simulink model "BD_DynamicCompareSims2"  (Simulink 4.1.1)
settings: Solver=VariableStepDiscrete  StartTime=0.0  StopTime=inf  FixedStep=1  RelTol=1e-3
undefined symbols (not defined in the file or in its folder): ALTIAHOME, cyc_mph_r1, ess_pwr_out_a1, ess_pwr_out_a2, ess_soc_hist1, ess_soc_hist2, fc_brake_trq1, fc_brake_trq2, fc_eff_out_a1, fc_eff_out_a2, fc_fuel_rate1, fc_fuel_rate2, fc_pwr_out_a1, fc_pwr_out_a2, fc_spd_est1, fc_spd_est2, gal1, gal2, gc_pwr_out_a1, gc_pwr_out_a2, gear_number1, gear_number2, grade1, grade2, mc_spd_out_a1, mc_spd_out_a2, mc_trq_out_a1, mc_trq_out_a2, mpha1, mpha2, time1, time2, trace_miss1, trace_miss2, veh_pwr_accel_a1, veh_pwr_accel_a2, veh_pwr_ascent_a1, veh_pwr_ascent_a2, veh_pwr_drag_a1, veh_pwr_drag_a2, veh_pwr_rr_a1, veh_pwr_rr_a2
libraries: simulink3 x4
settings Model: LastModifiedBy=abrooker

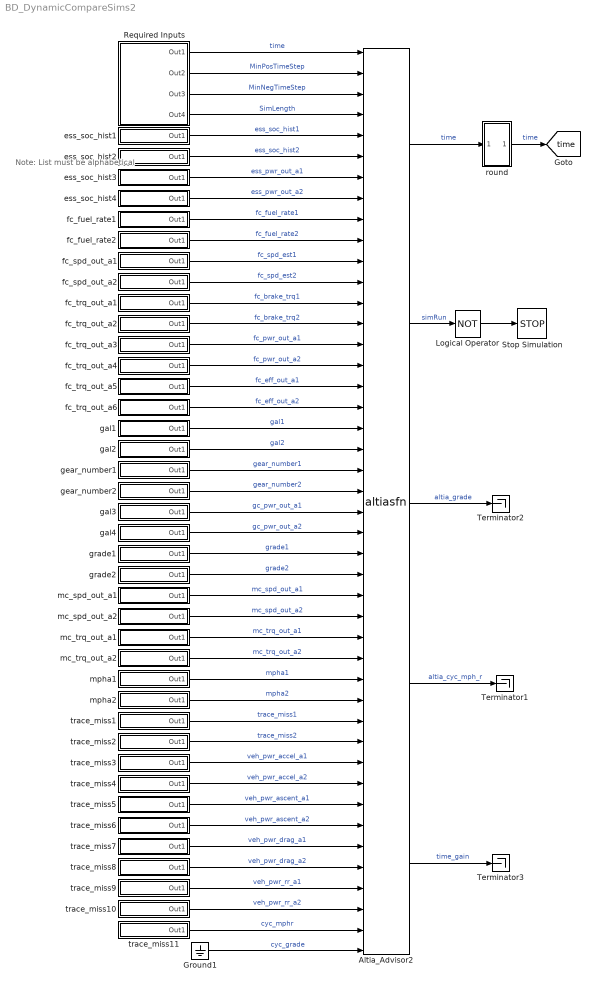
== system BD_DynamicCompareSims2 ==
  note: Note:  List must
      | be alphabetical
  Altia_Advisor2 : S-Function  FunctionName=altiasfn  Parameters=NumAltiaSfnInputs,NumAltiaSfnOutputs,ALTIAHOME  PortCounts=[]  SFunctionModules=libsdde.lib user32.lib  mask{NumAltiaSfnInputs=44, NumAltiaSfnOutputs=5}
      mask prompts: NumAltiaSfnInputs "Inputs to Altia S-Function:"; NumAltiaSfnOutputs "Outputs to Altia S-Function:"
      mask help: This block allows you to connect your signals to an Altia Design file. Specify the number of Inputs and Outputs you would like the Altia block to have (each line connected to the block can only be ONE signal wide ... no muxing into the Altia block).
      mask init:
      | altiahome
      settings: OpenFcn=AltiaClk
      mask Help: The first box is the number of inputs to the Altia S-Function.  The second box is the number of ouputs for the Altia S-Function.
      mask Display: disp('A L T I A')
  Ground1 : Ground
  Logical Operator : Logic  Operator=NOT  Inputs=2
  Required Inputs : Subsystem
      settings: RTWFcnNameOpts=Auto  RTWFileNameOpts=Auto
      mask Display: disp('Required Inputs');
  Stop Simulation : Stop
  Terminator1 : Terminator
  Terminator2 : Terminator
  Terminator3 : Terminator
  ess_soc_hist1 : Subsystem  mask{outputVector=ess_soc_hist1, timeVector=time1}
      mask prompts: outputVector "Output"; timeVector "Time Vector"
      settings: RTWFcnNameOpts=Auto  RTWFileNameOpts=Auto
      mask Display: disp('');
  ess_soc_hist2 : Subsystem  mask{outputVector=ess_soc_hist2, timeVector=time2}
      mask prompts: outputVector "Output"; timeVector "Time Vector"
      settings: RTWFcnNameOpts=Auto  RTWFileNameOpts=Auto
      mask Display: disp('');
  ess_soc_hist3 : Subsystem  mask{outputVector=ess_pwr_out_a1, timeVector=time1}
      mask prompts: outputVector "Output"; timeVector "Time Vector"
      settings: RTWFcnNameOpts=Auto  RTWFileNameOpts=Auto
      mask Display: disp('');
  ess_soc_hist4 : Subsystem  mask{outputVector=ess_pwr_out_a2, timeVector=time2}
      mask prompts: outputVector "Output"; timeVector "Time Vector"
      settings: RTWFcnNameOpts=Auto  RTWFileNameOpts=Auto
      mask Display: disp('');
  fc_fuel_rate1 : Subsystem  mask{outputVector=fc_fuel_rate1, timeVector=time1}
      mask prompts: outputVector "Output"; timeVector "Time Vector"
      settings: RTWFcnNameOpts=Auto  RTWFileNameOpts=Auto
      mask Display: disp('');
  fc_fuel_rate2 : Subsystem  mask{outputVector=fc_fuel_rate2, timeVector=time2}
      mask prompts: outputVector "Output"; timeVector "Time Vector"
      settings: RTWFcnNameOpts=Auto  RTWFileNameOpts=Auto
      mask Display: disp('');
  fc_spd_out_a1 : Subsystem  mask{outputVector=fc_spd_est1, timeVector=time1}
      mask prompts: outputVector "Output"; timeVector "Time Vector"
      settings: RTWFcnNameOpts=Auto  RTWFileNameOpts=Auto
      mask Display: disp('');
  fc_spd_out_a2 : Subsystem  mask{outputVector=fc_spd_est2, timeVector=time2}
      mask prompts: outputVector "Output"; timeVector "Time Vector"
      settings: RTWFcnNameOpts=Auto  RTWFileNameOpts=Auto
      mask Display: disp('');
  fc_trq_out_a1 : Subsystem  mask{outputVector=fc_brake_trq1, timeVector=time1}
      mask prompts: outputVector "Output"; timeVector "Time Vector"
      settings: RTWFcnNameOpts=Auto  RTWFileNameOpts=Auto
      mask Display: disp('');
  fc_trq_out_a2 : Subsystem  mask{outputVector=fc_brake_trq2, timeVector=time2}
      mask prompts: outputVector "Output"; timeVector "Time Vector"
      settings: RTWFcnNameOpts=Auto  RTWFileNameOpts=Auto
      mask Display: disp('');
  fc_trq_out_a3 : Subsystem  mask{outputVector=fc_pwr_out_a1, timeVector=time1}
      mask prompts: outputVector "Output"; timeVector "Time Vector"
      settings: RTWFcnNameOpts=Auto  RTWFileNameOpts=Auto
      mask Display: disp('');
  fc_trq_out_a4 : Subsystem  mask{outputVector=fc_pwr_out_a2, timeVector=time2}
      mask prompts: outputVector "Output"; timeVector "Time Vector"
      settings: RTWFcnNameOpts=Auto  RTWFileNameOpts=Auto
      mask Display: disp('');
  fc_trq_out_a5 : Subsystem  mask{outputVector=fc_eff_out_a1, timeVector=time1}
      mask prompts: outputVector "Output"; timeVector "Time Vector"
      settings: RTWFcnNameOpts=Auto  RTWFileNameOpts=Auto
      mask Display: disp('');
  fc_trq_out_a6 : Subsystem  mask{outputVector=fc_eff_out_a2, timeVector=time2}
      mask prompts: outputVector "Output"; timeVector "Time Vector"
      settings: RTWFcnNameOpts=Auto  RTWFileNameOpts=Auto
      mask Display: disp('');
  gal1 : Subsystem  mask{outputVector=gal1, timeVector=time1}
      mask prompts: outputVector "Output"; timeVector "Time Vector"
      settings: RTWFcnNameOpts=Auto  RTWFileNameOpts=Auto
      mask Display: disp('');
  gal2 : Subsystem  mask{outputVector=gal2, timeVector=time2}
      mask prompts: outputVector "Output"; timeVector "Time Vector"
      settings: RTWFcnNameOpts=Auto  RTWFileNameOpts=Auto
      mask Display: disp('');
  gal3 : Subsystem  mask{outputVector=gc_pwr_out_a1, timeVector=time1}
      mask prompts: outputVector "Output"; timeVector "Time Vector"
      settings: RTWFcnNameOpts=Auto  RTWFileNameOpts=Auto
      mask Display: disp('');
  gal4 : Subsystem  mask{outputVector=gc_pwr_out_a2, timeVector=time2}
      mask prompts: outputVector "Output"; timeVector "Time Vector"
      settings: RTWFcnNameOpts=Auto  RTWFileNameOpts=Auto
      mask Display: disp('');
  gear_number1 : Subsystem  mask{outputVector=gear_number1, timeVector=time1}
      mask prompts: outputVector "Output"; timeVector "Time Vector"
      settings: RTWFcnNameOpts=Auto  RTWFileNameOpts=Auto
      mask Display: disp('');
  gear_number2 : Subsystem  mask{outputVector=gear_number2, timeVector=time2}
      mask prompts: outputVector "Output"; timeVector "Time Vector"
      settings: RTWFcnNameOpts=Auto  RTWFileNameOpts=Auto
      mask Display: disp('');
  grade1 : Subsystem  mask{outputVector=grade1, timeVector=time1}
      mask prompts: outputVector "Output"; timeVector "Time Vector"
      settings: RTWFcnNameOpts=Auto  RTWFileNameOpts=Auto
      mask Display: disp('');
  grade2 : Subsystem  mask{outputVector=grade2, timeVector=time2}
      mask prompts: outputVector "Output"; timeVector "Time Vector"
      settings: RTWFcnNameOpts=Auto  RTWFileNameOpts=Auto
      mask Display: disp('');
  mc_spd_out_a1 : Subsystem  mask{outputVector=mc_spd_out_a1, timeVector=time1}
      mask prompts: outputVector "Output"; timeVector "Time Vector"
      settings: RTWFcnNameOpts=Auto  RTWFileNameOpts=Auto
      mask Display: disp('');
  mc_spd_out_a2 : Subsystem  mask{outputVector=mc_spd_out_a2, timeVector=time2}
      mask prompts: outputVector "Output"; timeVector "Time Vector"
      settings: RTWFcnNameOpts=Auto  RTWFileNameOpts=Auto
      mask Display: disp('');
  mc_trq_out_a1 : Subsystem  mask{outputVector=mc_trq_out_a1, timeVector=time1}
      mask prompts: outputVector "Output"; timeVector "Time Vector"
      settings: RTWFcnNameOpts=Auto  RTWFileNameOpts=Auto
      mask Display: disp('');
  mc_trq_out_a2 : Subsystem  mask{outputVector=mc_trq_out_a2, timeVector=time2}
      mask prompts: outputVector "Output"; timeVector "Time Vector"
      settings: RTWFcnNameOpts=Auto  RTWFileNameOpts=Auto
      mask Display: disp('');
  mpha1 : Subsystem  mask{outputVector=mpha1, timeVector=time1}
      mask prompts: outputVector "Output"; timeVector "Time Vector"
      settings: RTWFcnNameOpts=Auto  RTWFileNameOpts=Auto
      mask Display: disp('');
  mpha2 : Subsystem  mask{outputVector=mpha2, timeVector=time2}
      mask prompts: outputVector "Output"; timeVector "Time Vector"
      settings: RTWFcnNameOpts=Auto  RTWFileNameOpts=Auto
      mask Display: disp('');
  round : Subsystem  mask{DecPlace=.001}
      mask prompts: DecPlace "Decimal Place (Example:  .001 rounds 1.2222 to 1.2200)"
      settings: RTWFcnNameOpts=Auto  RTWFileNameOpts=Auto
  trace_miss1 : Subsystem  mask{outputVector=trace_miss1, timeVector=time1}
      mask prompts: outputVector "Output"; timeVector "Time Vector"
      settings: RTWFcnNameOpts=Auto  RTWFileNameOpts=Auto
      mask Display: disp('');
  trace_miss10 : Subsystem  mask{outputVector=veh_pwr_rr_a2, timeVector=time2}
      mask prompts: outputVector "Output"; timeVector "Time Vector"
      settings: RTWFcnNameOpts=Auto  RTWFileNameOpts=Auto
      mask Display: disp('');
  trace_miss11 : Subsystem  mask{outputVector=cyc_mph_r1, timeVector=time1}
      mask prompts: outputVector "Output"; timeVector "Time Vector"
      settings: RTWFcnNameOpts=Auto  RTWFileNameOpts=Auto
      mask Display: disp('');
  trace_miss2 : Subsystem  mask{outputVector=trace_miss2, timeVector=time2}
      mask prompts: outputVector "Output"; timeVector "Time Vector"
      settings: RTWFcnNameOpts=Auto  RTWFileNameOpts=Auto
      mask Display: disp('');
  trace_miss3 : Subsystem  mask{outputVector=veh_pwr_accel_a1, timeVector=time1}
      mask prompts: outputVector "Output"; timeVector "Time Vector"
      settings: RTWFcnNameOpts=Auto  RTWFileNameOpts=Auto
      mask Display: disp('');
  trace_miss4 : Subsystem  mask{outputVector=veh_pwr_accel_a2, timeVector=time2}
      mask prompts: outputVector "Output"; timeVector "Time Vector"
      settings: RTWFcnNameOpts=Auto  RTWFileNameOpts=Auto
      mask Display: disp('');
  trace_miss5 : Subsystem  mask{outputVector=veh_pwr_ascent_a1, timeVector=time1}
      mask prompts: outputVector "Output"; timeVector "Time Vector"
      settings: RTWFcnNameOpts=Auto  RTWFileNameOpts=Auto
      mask Display: disp('');
  trace_miss6 : Subsystem  mask{outputVector=veh_pwr_ascent_a2, timeVector=time2}
      mask prompts: outputVector "Output"; timeVector "Time Vector"
      settings: RTWFcnNameOpts=Auto  RTWFileNameOpts=Auto
      mask Display: disp('');
  trace_miss7 : Subsystem  mask{outputVector=veh_pwr_drag_a1, timeVector=time1}
      mask prompts: outputVector "Output"; timeVector "Time Vector"
      settings: RTWFcnNameOpts=Auto  RTWFileNameOpts=Auto
      mask Display: disp('');
  trace_miss8 : Subsystem  mask{outputVector=veh_pwr_drag_a2, timeVector=time2}
      mask prompts: outputVector "Output"; timeVector "Time Vector"
      settings: RTWFcnNameOpts=Auto  RTWFileNameOpts=Auto
      mask Display: disp('');
  trace_miss9 : Subsystem  mask{outputVector=veh_pwr_rr_a1, timeVector=time1}
      mask prompts: outputVector "Output"; timeVector "Time Vector"
      settings: RTWFcnNameOpts=Auto  RTWFileNameOpts=Auto
      mask Display: disp('');
  tag scope: time=global
  wires:
  Altia_Advisor2/1 -> round/1(In1)  "time"
  Required Inputs/2(Out2) -> Altia_Advisor2/2  "MinPosTimeStep"
  Required Inputs/3(Out3) -> Altia_Advisor2/3  "MinNegTimeStep"
  Required Inputs/4(Out4) -> Altia_Advisor2/4  "SimLength"
  Required Inputs/1(Out1) -> Altia_Advisor2/1  "time"
  round/1(Out1) -> [time]  "time"
  Altia_Advisor2/2 -> Logical Operator/1  "simRun"
  ess_soc_hist1/1(Out1) -> Altia_Advisor2/5  "ess_soc_hist1"
  ess_soc_hist2/1(Out1) -> Altia_Advisor2/6  "ess_soc_hist2"
  fc_fuel_rate2/1(Out1) -> Altia_Advisor2/10  "fc_fuel_rate2"
  fc_spd_out_a1/1(Out1) -> Altia_Advisor2/11  "fc_spd_est1"
  fc_spd_out_a2/1(Out1) -> Altia_Advisor2/12  "fc_spd_est2"
  fc_trq_out_a1/1(Out1) -> Altia_Advisor2/13  "fc_brake_trq1"
  fc_trq_out_a2/1(Out1) -> Altia_Advisor2/14  "fc_brake_trq2"
  Altia_Advisor2/3 -> Terminator2/1  "altia_grade"
  Altia_Advisor2/4 -> Terminator1/1  "altia_cyc_mph_r"
  Altia_Advisor2/5 -> Terminator3/1  "time_gain"
  fc_trq_out_a3/1(Out1) -> Altia_Advisor2/15  "fc_pwr_out_a1"
  gal1/1(Out1) -> Altia_Advisor2/19  "gal1"
  gal2/1(Out1) -> Altia_Advisor2/20  "gal2"
  gear_number1/1(Out1) -> Altia_Advisor2/21  "gear_number1"
  gear_number2/1(Out1) -> Altia_Advisor2/22  "gear_number2"
  grade1/1(Out1) -> Altia_Advisor2/25  "grade1"
  grade2/1(Out1) -> Altia_Advisor2/26  "grade2"
  mc_spd_out_a1/1(Out1) -> Altia_Advisor2/27  "mc_spd_out_a1"
  mc_spd_out_a2/1(Out1) -> Altia_Advisor2/28  "mc_spd_out_a2"
  mc_trq_out_a1/1(Out1) -> Altia_Advisor2/29  "mc_trq_out_a1"
  mc_trq_out_a2/1(Out1) -> Altia_Advisor2/30  "mc_trq_out_a2"
  mpha1/1(Out1) -> Altia_Advisor2/31  "mpha1"
  mpha2/1(Out1) -> Altia_Advisor2/32  "mpha2"
  trace_miss1/1(Out1) -> Altia_Advisor2/33  "trace_miss1"
  trace_miss2/1(Out1) -> Altia_Advisor2/34  "trace_miss2"
  trace_miss11/1(Out1) -> Altia_Advisor2/43  "cyc_mphr"
  Ground1/1 -> Altia_Advisor2/44  "cyc_grade"
  fc_trq_out_a4/1(Out1) -> Altia_Advisor2/16  "fc_pwr_out_a2"
  fc_trq_out_a5/1(Out1) -> Altia_Advisor2/17  "fc_eff_out_a1"
  fc_trq_out_a6/1(Out1) -> Altia_Advisor2/18  "fc_eff_out_a2"
  fc_fuel_rate1/1(Out1) -> Altia_Advisor2/9  "fc_fuel_rate1"
  ess_soc_hist3/1(Out1) -> Altia_Advisor2/7  "ess_pwr_out_a1"
  ess_soc_hist4/1(Out1) -> Altia_Advisor2/8  "ess_pwr_out_a2"
  gal3/1(Out1) -> Altia_Advisor2/23  "gc_pwr_out_a1"
  gal4/1(Out1) -> Altia_Advisor2/24  "gc_pwr_out_a2"
  trace_miss4/1(Out1) -> Altia_Advisor2/36  "veh_pwr_accel_a2"
  trace_miss5/1(Out1) -> Altia_Advisor2/37  "veh_pwr_ascent_a1"
  trace_miss6/1(Out1) -> Altia_Advisor2/38  "veh_pwr_ascent_a2"
  trace_miss8/1(Out1) -> Altia_Advisor2/40  "veh_pwr_drag_a2"
  trace_miss9/1(Out1) -> Altia_Advisor2/41  "veh_pwr_rr_a1"
  trace_miss10/1(Out1) -> Altia_Advisor2/42  "veh_pwr_rr_a2"
  trace_miss7/1(Out1) -> Altia_Advisor2/39  "veh_pwr_drag_a1"
  trace_miss3/1(Out1) -> Altia_Advisor2/35  "veh_pwr_accel_a1"
  Logical Operator/1 -> Stop Simulation/1

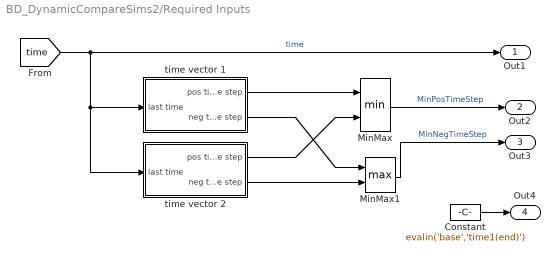
== system BD_DynamicCompareSims2/Required Inputs ==
  Constant : Constant  Value=evalin('base','time1(end)')
  MinMax : MinMax  Function=min  Inputs=2
  MinMax1 : MinMax  Function=max  Inputs=2
  time vector 1 : Subsystem  mask{time=evalin('base','time1')}
      mask prompts: time "Time Vector"
      settings: RTWFcnNameOpts=Auto  RTWFileNameOpts=Auto
  time vector 2 : Subsystem  mask{time=evalin('base','time2')}
      mask prompts: time "Time Vector"
      settings: RTWFcnNameOpts=Auto  RTWFileNameOpts=Auto
  Out1 : Outport  Port=1
  Out2 : Outport  Port=2
  Out3 : Outport  Port=3
  Out4 : Outport  Port=4
  wires:
  MinMax/1 -> Out2/1  "MinPosTimeStep"
  MinMax1/1 -> Out3/1  "MinNegTimeStep"
  time vector 1/1(pos time step) -> MinMax/1
  time vector 2/2(neg time step) -> MinMax1/2
  time vector 2/1(pos time step) -> MinMax/2
  time vector 1/2(neg time step) -> MinMax1/1
  [time] -> Out1/1, time vector 1/1(last time), time vector 2/1(last time)  "time"
  Constant/1 -> Out4/1

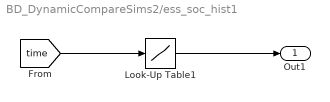
== system BD_DynamicCompareSims2/ess_soc_hist1 ==
  Look-Up Table1 : Lookup  InputValues=timeVector  OutputValues=outputVector
  Out1 : Outport  Port=1
  wires:
  [time] -> Look-Up Table1/1
  Look-Up Table1/1 -> Out1/1

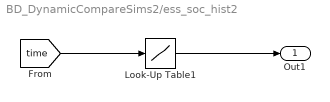
== system BD_DynamicCompareSims2/ess_soc_hist2 ==
  Look-Up Table1 : Lookup  InputValues=timeVector  OutputValues=outputVector
  Out1 : Outport  Port=1
  wires:
  [time] -> Look-Up Table1/1
  Look-Up Table1/1 -> Out1/1

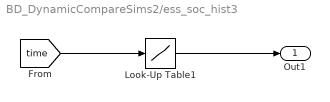
== system BD_DynamicCompareSims2/ess_soc_hist3 ==
  Look-Up Table1 : Lookup  InputValues=timeVector  OutputValues=outputVector
  Out1 : Outport  Port=1
  wires:
  Look-Up Table1/1 -> Out1/1
  [time] -> Look-Up Table1/1

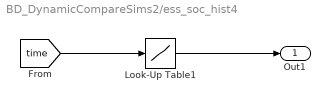
== system BD_DynamicCompareSims2/ess_soc_hist4 ==
  Look-Up Table1 : Lookup  InputValues=timeVector  OutputValues=outputVector
  Out1 : Outport  Port=1
  wires:
  Look-Up Table1/1 -> Out1/1
  [time] -> Look-Up Table1/1

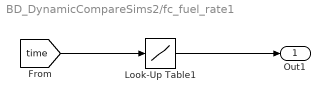
== system BD_DynamicCompareSims2/fc_fuel_rate1 ==
  Look-Up Table1 : Lookup  InputValues=timeVector  OutputValues=outputVector
  Out1 : Outport  Port=1
  wires:
  [time] -> Look-Up Table1/1
  Look-Up Table1/1 -> Out1/1

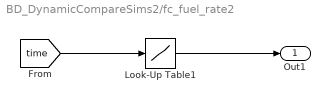
== system BD_DynamicCompareSims2/fc_fuel_rate2 ==
  Look-Up Table1 : Lookup  InputValues=timeVector  OutputValues=outputVector
  Out1 : Outport  Port=1
  wires:
  [time] -> Look-Up Table1/1
  Look-Up Table1/1 -> Out1/1

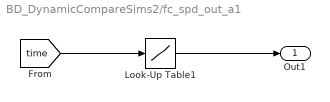
== system BD_DynamicCompareSims2/fc_spd_out_a1 ==
  Look-Up Table1 : Lookup  InputValues=timeVector  OutputValues=outputVector
  Out1 : Outport  Port=1
  wires:
  [time] -> Look-Up Table1/1
  Look-Up Table1/1 -> Out1/1

== system BD_DynamicCompareSims2/fc_spd_out_a2 ==
  Look-Up Table1 : Lookup  InputValues=timeVector  OutputValues=outputVector
  Out1 : Outport  Port=1
  wires:
  [time] -> Look-Up Table1/1
  Look-Up Table1/1 -> Out1/1

== system BD_DynamicCompareSims2/fc_trq_out_a1 ==
  Look-Up Table1 : Lookup  InputValues=timeVector  OutputValues=outputVector
  Out1 : Outport  Port=1
  wires:
  [time] -> Look-Up Table1/1
  Look-Up Table1/1 -> Out1/1

== system BD_DynamicCompareSims2/fc_trq_out_a2 ==
  Look-Up Table1 : Lookup  InputValues=timeVector  OutputValues=outputVector
  Out1 : Outport  Port=1
  wires:
  [time] -> Look-Up Table1/1
  Look-Up Table1/1 -> Out1/1

== system BD_DynamicCompareSims2/fc_trq_out_a3 ==
  Look-Up Table1 : Lookup  InputValues=timeVector  OutputValues=outputVector
  Out1 : Outport  Port=1
  wires:
  Look-Up Table1/1 -> Out1/1
  [time] -> Look-Up Table1/1

== system BD_DynamicCompareSims2/fc_trq_out_a4 ==
  Look-Up Table1 : Lookup  InputValues=timeVector  OutputValues=outputVector
  Out1 : Outport  Port=1
  wires:
  Look-Up Table1/1 -> Out1/1
  [time] -> Look-Up Table1/1

== system BD_DynamicCompareSims2/fc_trq_out_a5 ==
  Look-Up Table1 : Lookup  InputValues=timeVector  OutputValues=outputVector
  Out1 : Outport  Port=1
  wires:
  [time] -> Look-Up Table1/1
  Look-Up Table1/1 -> Out1/1

== system BD_DynamicCompareSims2/fc_trq_out_a6 ==
  Look-Up Table1 : Lookup  InputValues=timeVector  OutputValues=outputVector
  Out1 : Outport  Port=1
  wires:
  Look-Up Table1/1 -> Out1/1
  [time] -> Look-Up Table1/1

== system BD_DynamicCompareSims2/gal1 ==
  Look-Up Table1 : Lookup  InputValues=timeVector  OutputValues=outputVector
  Out1 : Outport  Port=1
  wires:
  [time] -> Look-Up Table1/1
  Look-Up Table1/1 -> Out1/1

== system BD_DynamicCompareSims2/gal2 ==
  Look-Up Table1 : Lookup  InputValues=timeVector  OutputValues=outputVector
  Out1 : Outport  Port=1
  wires:
  [time] -> Look-Up Table1/1
  Look-Up Table1/1 -> Out1/1

== system BD_DynamicCompareSims2/gal3 ==
  Look-Up Table1 : Lookup  InputValues=timeVector  OutputValues=outputVector
  Out1 : Outport  Port=1
  wires:
  Look-Up Table1/1 -> Out1/1
  [time] -> Look-Up Table1/1

== system BD_DynamicCompareSims2/gal4 ==
  Look-Up Table1 : Lookup  InputValues=timeVector  OutputValues=outputVector
  Out1 : Outport  Port=1
  wires:
  Look-Up Table1/1 -> Out1/1
  [time] -> Look-Up Table1/1

== system BD_DynamicCompareSims2/gear_number1 ==
  Look-Up Table1 : Lookup  InputValues=timeVector  OutputValues=outputVector
  Out1 : Outport  Port=1
  wires:
  [time] -> Look-Up Table1/1
  Look-Up Table1/1 -> Out1/1

== system BD_DynamicCompareSims2/gear_number2 ==
  Look-Up Table1 : Lookup  InputValues=timeVector  OutputValues=outputVector
  Out1 : Outport  Port=1
  wires:
  [time] -> Look-Up Table1/1
  Look-Up Table1/1 -> Out1/1

== system BD_DynamicCompareSims2/grade1 ==
  Look-Up Table1 : Lookup  InputValues=timeVector  OutputValues=outputVector
  Out1 : Outport  Port=1
  wires:
  [time] -> Look-Up Table1/1
  Look-Up Table1/1 -> Out1/1

== system BD_DynamicCompareSims2/grade2 ==
  Look-Up Table1 : Lookup  InputValues=timeVector  OutputValues=outputVector
  Out1 : Outport  Port=1
  wires:
  [time] -> Look-Up Table1/1
  Look-Up Table1/1 -> Out1/1

== system BD_DynamicCompareSims2/mc_spd_out_a1 ==
  Look-Up Table1 : Lookup  InputValues=timeVector  OutputValues=outputVector
  Out1 : Outport  Port=1
  wires:
  [time] -> Look-Up Table1/1
  Look-Up Table1/1 -> Out1/1

== system BD_DynamicCompareSims2/mc_spd_out_a2 ==
  Look-Up Table1 : Lookup  InputValues=timeVector  OutputValues=outputVector
  Out1 : Outport  Port=1
  wires:
  [time] -> Look-Up Table1/1
  Look-Up Table1/1 -> Out1/1

== system BD_DynamicCompareSims2/mc_trq_out_a1 ==
  Look-Up Table1 : Lookup  InputValues=timeVector  OutputValues=outputVector
  Out1 : Outport  Port=1
  wires:
  [time] -> Look-Up Table1/1
  Look-Up Table1/1 -> Out1/1

== system BD_DynamicCompareSims2/mc_trq_out_a2 ==
  Look-Up Table1 : Lookup  InputValues=timeVector  OutputValues=outputVector
  Out1 : Outport  Port=1
  wires:
  [time] -> Look-Up Table1/1
  Look-Up Table1/1 -> Out1/1

== system BD_DynamicCompareSims2/mpha1 ==
  Look-Up Table1 : Lookup  InputValues=timeVector  OutputValues=outputVector
  Out1 : Outport  Port=1
  wires:
  [time] -> Look-Up Table1/1
  Look-Up Table1/1 -> Out1/1

== system BD_DynamicCompareSims2/mpha2 ==
  Look-Up Table1 : Lookup  InputValues=timeVector  OutputValues=outputVector
  Out1 : Outport  Port=1
  wires:
  [time] -> Look-Up Table1/1
  Look-Up Table1/1 -> Out1/1

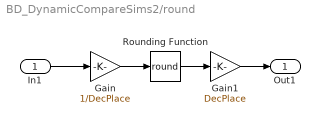
== system BD_DynamicCompareSims2/round ==
  In1 : Inport  Port=1  LatchInput=off
  Gain : Gain  Gain=1/DecPlace  Multiplication=Element-wise(K.*u)  SaturateOnIntegerOverflow=on
  Gain1 : Gain  Gain=DecPlace  Multiplication=Element-wise(K.*u)  SaturateOnIntegerOverflow=on
  Rounding Function : Rounding  Operator=round
  Out1 : Outport  Port=1
  wires:
  Rounding Function/1 -> Gain1/1
  Gain/1 -> Rounding Function/1
  In1/1 -> Gain/1
  Gain1/1 -> Out1/1

== system BD_DynamicCompareSims2/trace_miss1 ==
  Look-Up Table1 : Lookup  InputValues=timeVector  OutputValues=outputVector
  Out1 : Outport  Port=1
  wires:
  [time] -> Look-Up Table1/1
  Look-Up Table1/1 -> Out1/1

== system BD_DynamicCompareSims2/trace_miss10 ==
  Look-Up Table1 : Lookup  InputValues=timeVector  OutputValues=outputVector
  Out1 : Outport  Port=1
  wires:
  Look-Up Table1/1 -> Out1/1
  [time] -> Look-Up Table1/1

== system BD_DynamicCompareSims2/trace_miss11 ==
  Look-Up Table1 : Lookup  InputValues=timeVector  OutputValues=outputVector
  Out1 : Outport  Port=1
  wires:
  [time] -> Look-Up Table1/1
  Look-Up Table1/1 -> Out1/1

== system BD_DynamicCompareSims2/trace_miss2 ==
  Look-Up Table1 : Lookup  InputValues=timeVector  OutputValues=outputVector
  Out1 : Outport  Port=1
  wires:
  [time] -> Look-Up Table1/1
  Look-Up Table1/1 -> Out1/1

== system BD_DynamicCompareSims2/trace_miss3 ==
  Look-Up Table1 : Lookup  InputValues=timeVector  OutputValues=outputVector
  Out1 : Outport  Port=1
  wires:
  Look-Up Table1/1 -> Out1/1
  [time] -> Look-Up Table1/1

== system BD_DynamicCompareSims2/trace_miss4 ==
  Look-Up Table1 : Lookup  InputValues=timeVector  OutputValues=outputVector
  Out1 : Outport  Port=1
  wires:
  Look-Up Table1/1 -> Out1/1
  [time] -> Look-Up Table1/1

== system BD_DynamicCompareSims2/trace_miss5 ==
  Look-Up Table1 : Lookup  InputValues=timeVector  OutputValues=outputVector
  Out1 : Outport  Port=1
  wires:
  [time] -> Look-Up Table1/1
  Look-Up Table1/1 -> Out1/1

== system BD_DynamicCompareSims2/trace_miss6 ==
  Look-Up Table1 : Lookup  InputValues=timeVector  OutputValues=outputVector
  Out1 : Outport  Port=1
  wires:
  [time] -> Look-Up Table1/1
  Look-Up Table1/1 -> Out1/1

== system BD_DynamicCompareSims2/trace_miss7 ==
  Look-Up Table1 : Lookup  InputValues=timeVector  OutputValues=outputVector
  Out1 : Outport  Port=1
  wires:
  [time] -> Look-Up Table1/1
  Look-Up Table1/1 -> Out1/1

== system BD_DynamicCompareSims2/trace_miss8 ==
  Look-Up Table1 : Lookup  InputValues=timeVector  OutputValues=outputVector
  Out1 : Outport  Port=1
  wires:
  [time] -> Look-Up Table1/1
  Look-Up Table1/1 -> Out1/1

== system BD_DynamicCompareSims2/trace_miss9 ==
  Look-Up Table1 : Lookup  InputValues=timeVector  OutputValues=outputVector
  Out1 : Outport  Port=1
  wires:
  Look-Up Table1/1 -> Out1/1
  [time] -> Look-Up Table1/1

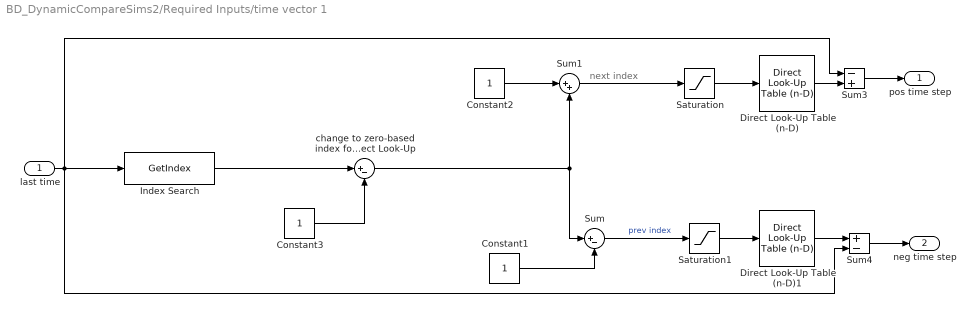
== system BD_DynamicCompareSims2/Required Inputs/time vector 1 ==
  note: next index
  last time : Inport  Port=1  LatchInput=off
  Constant1 : Constant  Value=1
  Constant2 : Constant  Value=1
  Constant3 : Constant  Value=1
  Direct Look-Up Table (n-D) : simulink3/Functions & Tables/Direct Look-Up Table (n-D)  maskTabDims=1  explicitNumDims=1  outDims=Element  tabIsInput=off  mxTable=time  clipFlag=None
  Direct Look-Up Table (n-D)1 : simulink3/Functions & Tables/Direct Look-Up Table (n-D)  maskTabDims=1  explicitNumDims=1  outDims=Element  tabIsInput=off  mxTable=time  clipFlag=None
  Index Search : S-Function  FunctionName=GetIndex  Parameters=time  PortCounts=[]  SFunctionModules=''
  Saturation : Saturate  UpperLimit=length(time)  LowerLimit=0  LinearizeAsGain=on
  Saturation1 : Saturate  UpperLimit=length(time)  LowerLimit=0  LinearizeAsGain=on
  Sum : Sum  Inputs=|+-  SaturateOnIntegerOverflow=on
  Sum1 : Sum  Inputs=|++  SaturateOnIntegerOverflow=on
  Sum3 : Sum  Inputs=-+  SaturateOnIntegerOverflow=on
  Sum4 : Sum  Inputs=+-  SaturateOnIntegerOverflow=on
  change to zero-based index for Direct Look-Up : Sum  Inputs=|+-  SaturateOnIntegerOverflow=on
  pos time step : Outport  Port=1
  neg time step : Outport  Port=2
  wires:
  Sum4/1 -> neg time step/1
  Direct Look-Up Table (n-D)1/1 -> Sum4/1
  Direct Look-Up Table (n-D)/1 -> Sum3/2
  Sum3/1 -> pos time step/1
  last time/1 -> Index Search/1, Sum3/1, Sum4/2
  Saturation1/1 -> Direct Look-Up Table (n-D)1/1
  Saturation/1 -> Direct Look-Up Table (n-D)/1
  Sum1/1 -> Saturation/1
  Constant2/1 -> Sum1/1
  Constant1/1 -> Sum/2
  Sum/1 -> Saturation1/1  "prev index"
  Index Search/1 -> change to zero-based index for Direct Look-Up/1
  change to zero-based index for Direct Look-Up/1 -> Sum1/2, Sum/1
  Constant3/1 -> change to zero-based index for Direct Look-Up/2

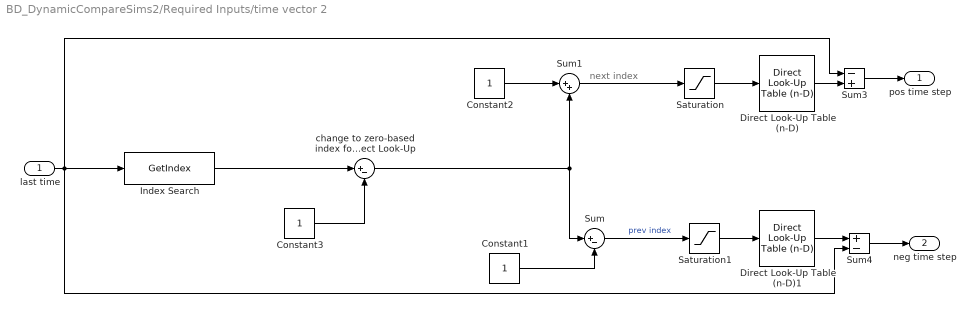
== system BD_DynamicCompareSims2/Required Inputs/time vector 2 ==
  note: next index
  last time : Inport  Port=1  LatchInput=off
  Constant1 : Constant  Value=1
  Constant2 : Constant  Value=1
  Constant3 : Constant  Value=1
  Direct Look-Up Table (n-D) : simulink3/Functions & Tables/Direct Look-Up Table (n-D)  maskTabDims=1  explicitNumDims=1  outDims=Element  tabIsInput=off  mxTable=time  clipFlag=None
  Direct Look-Up Table (n-D)1 : simulink3/Functions & Tables/Direct Look-Up Table (n-D)  maskTabDims=1  explicitNumDims=1  outDims=Element  tabIsInput=off  mxTable=time  clipFlag=None
  Index Search : S-Function  FunctionName=GetIndex  Parameters=time  PortCounts=[]  SFunctionModules=''
  Saturation : Saturate  UpperLimit=length(time)  LowerLimit=0  LinearizeAsGain=on
  Saturation1 : Saturate  UpperLimit=length(time)  LowerLimit=0  LinearizeAsGain=on
  Sum : Sum  Inputs=|+-  SaturateOnIntegerOverflow=on
  Sum1 : Sum  Inputs=|++  SaturateOnIntegerOverflow=on
  Sum3 : Sum  Inputs=-+  SaturateOnIntegerOverflow=on
  Sum4 : Sum  Inputs=+-  SaturateOnIntegerOverflow=on
  change to zero-based index for Direct Look-Up : Sum  Inputs=|+-  SaturateOnIntegerOverflow=on
  pos time step : Outport  Port=1
  neg time step : Outport  Port=2
  wires:
  Constant3/1 -> change to zero-based index for Direct Look-Up/2
  change to zero-based index for Direct Look-Up/1 -> Sum/1, Sum1/2
  Index Search/1 -> change to zero-based index for Direct Look-Up/1
  Sum/1 -> Saturation1/1  "prev index"
  Constant1/1 -> Sum/2
  Constant2/1 -> Sum1/1
  Sum1/1 -> Saturation/1
  Saturation/1 -> Direct Look-Up Table (n-D)/1
  Saturation1/1 -> Direct Look-Up Table (n-D)1/1
  last time/1 -> Sum4/2, Sum3/1, Index Search/1
  Sum3/1 -> pos time step/1
  Direct Look-Up Table (n-D)/1 -> Sum3/2
  Direct Look-Up Table (n-D)1/1 -> Sum4/1
  Sum4/1 -> neg time step/1
